simulink model "lmsxyplot"  (Simulink 6.0)
settings: Solver=FixedStepDiscrete  StartTime=0.0  StopTime=1500  RelTol=1e-3
InitFcn:
  | w=[0.5 0.5 ones(1,18)];
  | z=zeros(1,18);
undefined symbols (not defined in the file or in its folder): lmsxy
libraries: simulink x5, dspsrcs4 x4, dspadpt3 x4, dsparch4 x1
settings Model: Creator=navan  LastModifiedBy=navan
settings DataIOCC: SignalLoggingName=sigsOut
settings DebuggingCC: CheckExecutionContextPreStartOutputMsg=on  CheckExecutionContextRuntimeOutputMsg=on  SolverPrmCheckMsg=none
settings HardwareCC: TargetUnknown=on
settings ModelReferenceCC: UpdateModelReferenceTargets=IfOutOfDate
settings GRTTargetCC: LifeSpan=inf
settings SFSimCC: SFSimApplyToAllLibs=on  SFSimBuildMode=Incremental

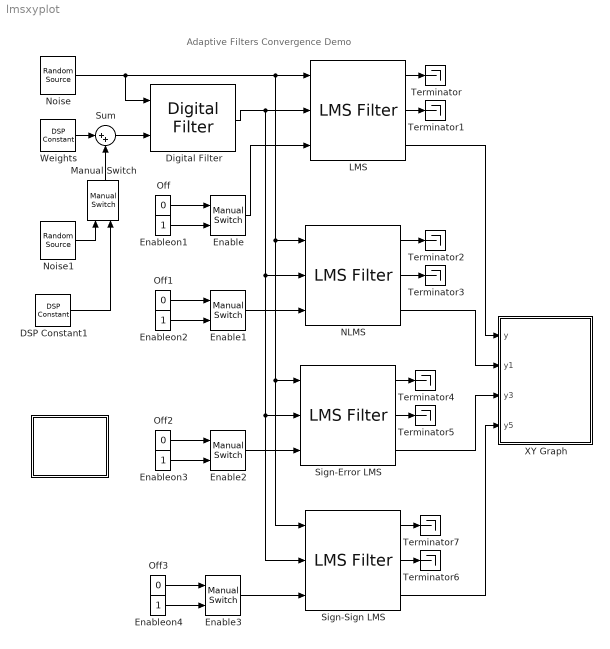
== system lmsxyplot ==
  note: Adaptive Filters Convergence Demo
  " " : Subsystem  EnableExecutionContextPropagation=on
      mask Type: Frame-Based Simulation Info
      mask Display: disp('Info')
  DSP Constant1 : dspsrcs4/DSP Constant  Value=0  SampleMode=Discrete  discreteOutput=Sample-based  continuousOutput=Sample-based  sampTime=1  framePeriod=2  dataType=Inherit from 'Constant value'  isSigned=on  wordLen=16  udDataType=sfix(16)  fracBitsMode=Best precision  numFracBits=15  InterpretAs1D=-inf  Ts=-inf  FramebasedOutput=-inf
  Digital Filter : dsparch4/Digital Filter  DialogController=dspDDGCreate  DialogControllerArgs=DataTag0  TypePopup=FIR (all zeros)  IIRFiltStruct=Direct form II transposed  AllPoleFiltStruct=Direct form  FIRFiltStruct=Direct form  CoeffSource=Input port(s)  NumCoeffs=[1 2]  DenCoeffs=[1 0.1]  BiQuadCoeffs=[1 0.3 0.4 1 0.1 0.2]  LatticeCoeffs=[0.2 0.4]  denIgnore=on  FiltPerSampPopup=One filter per frame  IC=0  ICnum=0  ICden=0  roundingMode=Floor  overflowMode=off  ScaleValues=0  scaleValueFracLength=14  tapSumFracLength=30  stageInFracLength=15  stageOutFracLength=15
  Enable{,1..3} (4 alike) : simulink/Signal Routing/Manual Switch  sw=0  action=0
  Enableon{1..4} (4 alike) : Constant  OutDataTypeMode=boolean
  LMS : dspadpt3/LMS Filter  DialogController=dspDDGCreate  DialogControllerArgs=DataTag1  Algo=LMS  L=20  stepflag=Dialog  mu=0.005  leakage=1.0  ic=[0 0 z]  Adapt=on  resetflag=None  weights=on  firstCoeffMode=User-defined  firstCoeffWordLength=16  firstCoeffFracLength=15  secondCoeffMode=User-defined  secondCoeffWordLength=2  secondCoeffFracLength=15  accumMode=User-defined  accumWordLength=32  accumFracLength=20  accum2Mode=User-defined  accum2FracLength=20  prodOutputMode=User-defined  prodOutputWordLength=32  prodOutputFracLength=20  prodOutput2Mode=User-defined  prodOutput2FracLength=20  prodOutput3Mode=User-defined  prodOutput3FracLength=20  prodOutput4Mode=User-defined  prodOutput4FracLength=20  quotientMode=User-defined  quotientFracLength=20  memoryMode=User-defined  memoryWordLength=16  memoryFracLength=15  roundingMode=Nearest  overflowMode=on
  Manual Switch : simulink/Signal Routing/Manual Switch  Orientation=up  sw=0  action=0
  NLMS : dspadpt3/LMS Filter  DialogController=dspDDGCreate  DialogControllerArgs=DataTag2  Algo=Normalized LMS  L=20  stepflag=Dialog  mu=0.05  leakage=1.0  ic=[1 0 z]  Adapt=on  resetflag=None  weights=on  firstCoeffMode=User-defined  firstCoeffWordLength=16  firstCoeffFracLength=15  secondCoeffMode=User-defined  secondCoeffWordLength=2  secondCoeffFracLength=15  accumMode=User-defined  accumWordLength=32  accumFracLength=20  accum2Mode=User-defined  accum2FracLength=20  prodOutputMode=User-defined  prodOutputWordLength=32  prodOutputFracLength=20  prodOutput2Mode=User-defined  prodOutput2FracLength=20  prodOutput3Mode=User-defined  prodOutput3FracLength=20  prodOutput4Mode=User-defined  prodOutput4FracLength=20  quotientMode=User-defined  quotientFracLength=20  memoryMode=User-defined  memoryWordLength=16  memoryFracLength=15  roundingMode=Nearest  overflowMode=on
  Noise : dspsrcs4/Random Source  SrcType=Gaussian  NormMethod=Ziggurat  CltLength=12  Min=0  Max=1  Mean=0  Var=1  RepMode=Specify seed  Seed=[23341]  Inherit=off  SampMode=Discrete  SampTime=1  SampFrame=1  DataType=Double  OutComplex=Real
  Noise1 : dspsrcs4/Random Source  SrcType=Gaussian  NormMethod=Ziggurat  CltLength=12  Min=0  Max=1  Mean=0  Var=0.01  RepMode=Specify seed  Seed=[23341]  Inherit=off  SampMode=Discrete  SampTime=1/20  SampFrame=20  DataType=Double  OutComplex=Real
  Off{,1..3} (4 alike) : Constant  Value=0  OutDataTypeMode=boolean
  Sign-Error LMS : dspadpt3/LMS Filter  DialogController=dspDDGCreate  DialogControllerArgs=DataTag3  Algo=Sign-Error LMS  L=20  stepflag=Dialog  mu=0.005  leakage=1.0  ic=[0 1 z]  Adapt=on  resetflag=None  weights=on  firstCoeffMode=User-defined  firstCoeffWordLength=16  firstCoeffFracLength=15  secondCoeffMode=User-defined  secondCoeffWordLength=2  secondCoeffFracLength=15  accumMode=User-defined  accumWordLength=32  accumFracLength=20  accum2Mode=User-defined  accum2FracLength=20  prodOutputMode=User-defined  prodOutputWordLength=32  prodOutputFracLength=20  prodOutput2Mode=User-defined  prodOutput2FracLength=20  prodOutput3Mode=User-defined  prodOutput3FracLength=20  prodOutput4Mode=User-defined  prodOutput4FracLength=20  quotientMode=User-defined  quotientFracLength=20  memoryMode=User-defined  memoryWordLength=16  memoryFracLength=15  roundingMode=Nearest  overflowMode=on
  Sign-Sign LMS : dspadpt3/LMS Filter  DialogController=dspDDGCreate  DialogControllerArgs=DataTag4  Algo=Sign-Sign LMS  L=20  stepflag=Dialog  mu=0.005  leakage=1.0  ic=[1 1 z]  Adapt=on  resetflag=None  weights=on  firstCoeffMode=User-defined  firstCoeffWordLength=16  firstCoeffFracLength=15  secondCoeffMode=User-defined  secondCoeffWordLength=2  secondCoeffFracLength=15  accumMode=User-defined  accumWordLength=32  accumFracLength=20  accum2Mode=User-defined  accum2FracLength=20  prodOutputMode=User-defined  prodOutputWordLength=32  prodOutputFracLength=20  prodOutput2Mode=User-defined  prodOutput2FracLength=20  prodOutput3Mode=User-defined  prodOutput3FracLength=20  prodOutput4Mode=User-defined  prodOutput4FracLength=20  quotientMode=User-defined  quotientFracLength=20  memoryMode=User-defined  memoryWordLength=16  memoryFracLength=15  roundingMode=Nearest  overflowMode=on
  Sum : Sum  Inputs=|++  SaturateOnIntegerOverflow=on
  Terminator{,1..7} (8 alike) : Terminator
  Weights : dspsrcs4/DSP Constant  Value=w'  SampleMode=Discrete  discreteOutput=Sample-based  continuousOutput=Sample-based  sampTime=1  framePeriod=2  dataType=Inherit from 'Constant value'  isSigned=on  wordLen=16  udDataType=sfix(16)  fracBitsMode=Best precision  numFracBits=15  InterpretAs1D=-inf  Ts=-inf  FramebasedOutput=-inf
  XY Graph : Subsystem  LoadFcn=lmsxy([],[],[],'LoadBlock',[])  StopFcn=lmsxy([],[],[],'Stop',[])  TreatAsAtomicUnit=on  EnableExecutionContextPropagation=on  SimViewingDevice=on  mask(XY scope.){xmin=0, xmax=1, ymin=0, ymax=1, st=-1, R=[0 1], W=w}
      mask prompts: xmin "x-min:"; xmax "x-max:"; ymin "y-min:"; ymax "y-max:"; st "Sample time:"; R "Input parameters [mean variance]"; W "Weights"
      mask help: XY scope using MATLAB graph window. First input is used as time base. Enter plotting ranges.
      mask init:
      | lmsxy([],[],[],'Start', [R W(1:2) xmin xmax ymin ymax])
      settings: CopyFcn=lmsxy([],[],[],'CopyBlock',[])  DeleteFcn=lmsxy([],[],[],'DeleteBlock',[])  NameChangeFcn=lmsxy([],[],[],'NameChange',[])
      mask Help: This block can be used to explore limit cycles. Look at the m-file sfunxy.m to see how it works.
      mask Display: plot([.05 .95 .95 .05 .05],[.45 .45 .95 .95 .45], 0.5+cos(0:0.1:2*pi)*0.3,0.7+sin(0:0.1:2*pi)*0.2)
  wires:
  Noise/1 -> LMS/1, NLMS/1, Sign-Error LMS/1, Sign-Sign LMS/1, Digital Filter/1
  Digital Filter/1 -> LMS/2, NLMS/2, Sign-Error LMS/2, Sign-Sign LMS/2
  LMS/1 -> Terminator/1
  LMS/2 -> Terminator1/1
  LMS/3 -> XY Graph/1(y)
  NLMS/3 -> XY Graph/2(y1)
  Sign-Error LMS/3 -> XY Graph/3(y3)
  NLMS/1 -> Terminator2/1
  NLMS/2 -> Terminator3/1
  Sign-Error LMS/1 -> Terminator4/1
  Sign-Error LMS/2 -> Terminator5/1
  Sign-Sign LMS/2 -> Terminator6/1
  Sign-Sign LMS/1 -> Terminator7/1
  Enable/1 -> LMS/3
  Enable1/1 -> NLMS/3
  Enable3/1 -> Sign-Sign LMS/3
  Sum/1 -> Digital Filter/2
  Weights/1 -> Sum/1
  Manual Switch/1 -> Sum/2
  Noise1/1 -> Manual Switch/1
  DSP Constant1/1 -> Manual Switch/2
  Off/1 -> Enable/1
  Enableon1/1 -> Enable/2
  Off1/1 -> Enable1/1
  Enableon2/1 -> Enable1/2
  Enable2/1 -> Sign-Error LMS/3
  Off2/1 -> Enable2/1
  Enableon3/1 -> Enable2/2
  Off3/1 -> Enable3/1
  Enableon4/1 -> Enable3/2
  Sign-Sign LMS/3 -> XY Graph/4(y5)

== system lmsxyplot/  ==
  note: Adaptive filter convergence
      |
      | This demo shows the convergence path taken by different adaptive filtering algorithms. The plot is a sequence
      | of points of the form (w1,w2) where w1 and w2 are the weights of the adaptive filter. The blue dots in the
      | figure indicate the contour lines of the error surface.
      |
      | Zoom(Tools->Zoom In) into the graph to see properties of convergence path.
      |
      | This demo does not depict the convergence speed of the different algorithms.
      | You can experiment with different step-size values for the adaptive filters to see the change in convergence paths.
      | Each of the adaptive filters can be enabled or disabled separately.
      |
      | LMS - Least mean square
      | NLMS - Normalized LMS
      | SELMS - Sign-error LMS
      | SSLMS - Sign-sign LMS

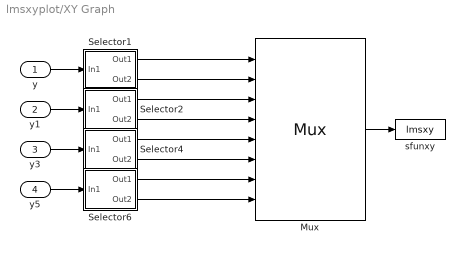
== system lmsxyplot/XY Graph ==
  y : Inport  LatchInput=off
  y1 : Inport  Port=2  LatchInput=off
  y3 : Inport  Port=3  LatchInput=off
  y5 : Inport  Port=4  LatchInput=off
  Mux : Mux  Inputs=8
  Selector1 : Subsystem  EnableExecutionContextPropagation=on
  Selector2 : Subsystem  EnableExecutionContextPropagation=on
  Selector4 : Subsystem  EnableExecutionContextPropagation=on
  Selector6 : Subsystem  EnableExecutionContextPropagation=on
  sfunxy : S-Function  FunctionName=lmsxy  Parameters=[xmin xmax ymin ymax 1:6], st
  wires:
  Selector1/2(Out2) -> Mux/2
  Mux/1 -> sfunxy/1
  Selector1/1(Out1) -> Mux/1
  Selector2/1(Out1) -> Mux/3
  Selector2/2(Out2) -> Mux/4
  Selector4/1(Out1) -> Mux/5
  Selector4/2(Out2) -> Mux/6
  Selector6/1(Out1) -> Mux/7
  Selector6/2(Out2) -> Mux/8
  y/1 -> Selector1/1(In1)
  y1/1 -> Selector2/1(In1)
  y3/1 -> Selector4/1(In1)
  y5/1 -> Selector6/1(In1)

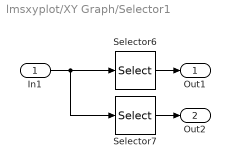
== system lmsxyplot/XY Graph/Selector1 ==
  In1 : Inport  LatchInput=off
  Selector6 : Selector  Elements=2
  Selector7 : Selector
  Out1 : Outport
  Out2 : Outport  Port=2
  wires:
  Selector7/1 -> Out2/1
  Selector6/1 -> Out1/1
  In1/1 -> Selector7/1, Selector6/1

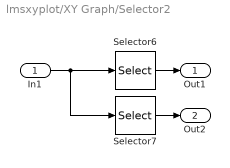
== system lmsxyplot/XY Graph/Selector2 ==
  In1 : Inport  LatchInput=off
  Selector6 : Selector  Elements=2
  Selector7 : Selector
  Out1 : Outport
  Out2 : Outport  Port=2
  wires:
  Selector7/1 -> Out2/1
  Selector6/1 -> Out1/1
  In1/1 -> Selector7/1, Selector6/1

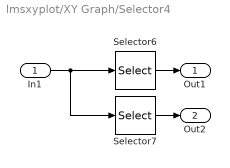
== system lmsxyplot/XY Graph/Selector4 ==
  In1 : Inport  LatchInput=off
  Selector6 : Selector  Elements=2
  Selector7 : Selector
  Out1 : Outport
  Out2 : Outport  Port=2
  wires:
  In1/1 -> Selector6/1, Selector7/1
  Selector6/1 -> Out1/1
  Selector7/1 -> Out2/1

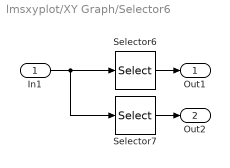
== system lmsxyplot/XY Graph/Selector6 ==
  In1 : Inport  LatchInput=off
  Selector6 : Selector  Elements=2
  Selector7 : Selector
  Out1 : Outport
  Out2 : Outport  Port=2
  wires:
  Selector7/1 -> Out2/1
  Selector6/1 -> Out1/1
  In1/1 -> Selector7/1, Selector6/1
